simulink model "exercitiul2"  (R2021b)
settings: Solver=VariableStepAuto  StartTime=0.0  StopTime=10.0  RelTol=1e-3
values from neighbouring files (symbols this model uses):
  A = [-1 0 0; -1 -2 -101; 1 1 0]    [exercitiul1.m]
  Ad1 = double(Ad)    [exercitiul1.m]
  B = [0 1; 1 -1; 0 0]    [exercitiul1.m]
  Bd1 = double(Bd)    [exercitiul1.m]
  C = [1 0 101]    [exercitiul1.m]
  Cd = C    [exercitiul1.m]
  D = [0 0]    [exercitiul1.m]
  Dd = D    [exercitiul1.m]
  h = 0.1    [exercitiul1.m]
undefined symbols (not defined in the file or in its folder): den1z, den2z, num1z, num2z
settings Model: Creator=george.tudor1906  LastModifiedBy=george.tudor1906

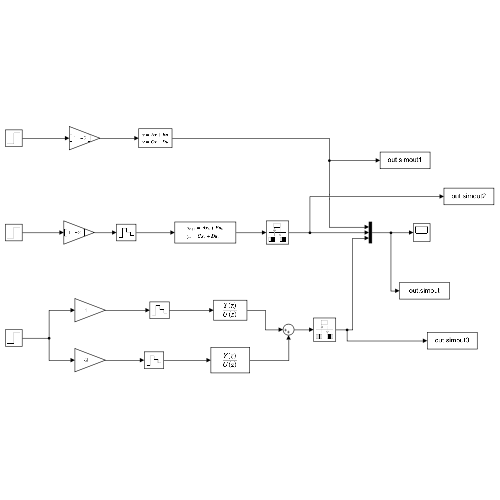
[thumbnail: Simulink's stored preview of the top-level diagram]
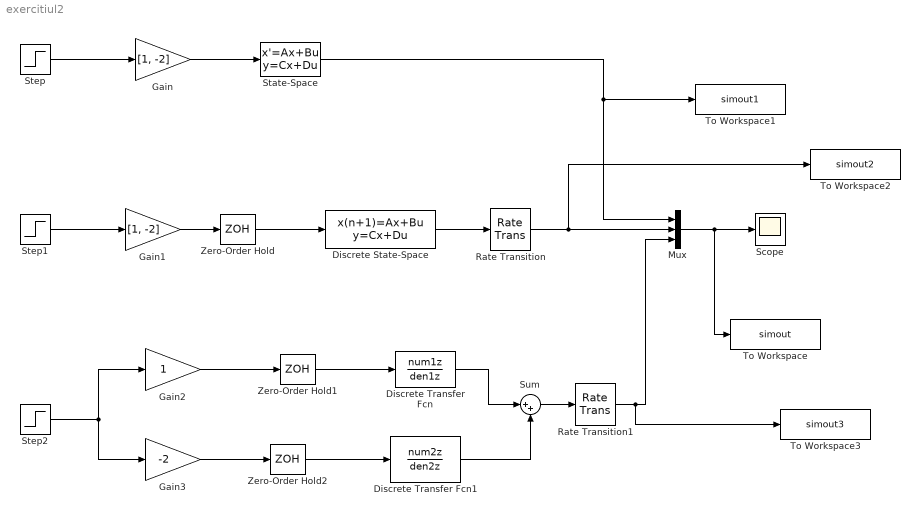
== system exercitiul2 ==
  Discrete Transfer Fcn : DiscreteTransferFcn  Numerator=num1z  Denominator=den1z
  Discrete Transfer Fcn1 : DiscreteTransferFcn  Numerator=num2z  Denominator=den2z
  Discrete State-Space : DiscreteStateSpace  A=Ad1  B=Bd1  C=Cd  D=Dd  SampleTime=-1
  Gain : Gain  Gain=[1, -2]
  Gain1 : Gain  Gain=[1, -2]
  Gain2 : Gain
  Gain3 : Gain  Gain=-2
  Mux : Mux  Inputs=3
  Rate Transition : RateTransition
  Rate Transition1 : RateTransition
  Scope : Scope
  State-Space : StateSpace  A=A  B=B  C=C  D=D  InitialCondition=0
  Step : Step  SampleTime=0
  Step1 : Step  SampleTime=0
  Step2 : Step  SampleTime=0
  Sum : Sum  Inputs=|++
  To Workspace : ToWorkspace  VariableName=simout  SaveFormat=Timeseries  SampleTime=-1
  To Workspace1 : ToWorkspace  VariableName=simout1  SaveFormat=Timeseries  SampleTime=-1
  To Workspace2 : ToWorkspace  VariableName=simout2  SaveFormat=Timeseries  SampleTime=-1
  To Workspace3 : ToWorkspace  VariableName=simout3  SaveFormat=Timeseries  SampleTime=-1
  Zero-Order Hold : ZeroOrderHold  SampleTime=h
  Zero-Order Hold1 : ZeroOrderHold  SampleTime=h
  Zero-Order Hold2 : ZeroOrderHold  SampleTime=h
  wires:
  Step/1 -> Gain/1
  Gain/1 -> State-Space/1
  Step1/1 -> Gain1/1
  Gain1/1 -> Zero-Order Hold/1
  Zero-Order Hold/1 -> Discrete State-Space/1
  Discrete State-Space/1 -> Rate Transition/1
  Gain2/1 -> Zero-Order Hold1/1
  Gain3/1 -> Zero-Order Hold2/1
  Zero-Order Hold1/1 -> Discrete Transfer Fcn/1
  Zero-Order Hold2/1 -> Discrete Transfer Fcn1/1
  Step2/1 -> Gain3/1, Gain2/1
  Discrete Transfer Fcn/1 -> Sum/1
  Discrete Transfer Fcn1/1 -> Sum/2
  Mux/1 -> To Workspace/1, Scope/1
  State-Space/1 -> To Workspace1/1, Mux/1
  Rate Transition/1 -> To Workspace2/1, Mux/2
  Sum/1 -> Rate Transition1/1
  Rate Transition1/1 -> To Workspace3/1, Mux/3
